simulink model "IDM_vs_DDM"  (R2014a)
settings: Solver=ode45  StartTime=0.0  StopTime=10.0  RelTol=1e-3
settings Model: Creator=Administrator  LastModifiedBy=Administrator

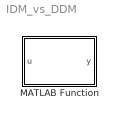
== system IDM_vs_DDM ==
  MATLAB Function : MATLAB Function  TreatAsAtomicUnit=on

== matlab function IDM_vs_DDM/MATLAB Function ==
  data: u input; y output
function y = fcn(u)
%#codegen

y = u;
